simulink model "ctrl_TT_ad_ctrl_cpp_ros_feedback"  (R2022b)
settings: Solver=FixedStepAuto  StartTime=0.0  StopTime=Tf  FixedStep=0.05  RelTol=1e-3
StopFcn:
  | save('testdata')
values from neighbouring files (symbols this model uses):
  adap = 1    [testdata.mat]
  Ba_0 = [0 0 0 0 0 0]    [testdata.mat]
  Bb = 4418825.3321    [testdata.mat]
  Bv_0 = [-5.14444 0 0 0 0 0]    [testdata.mat]
  Bx_0 = [70.34790039 -18.70597267 -370.8000183 0 0 0]    [testdata.mat]
  Cp = [-70.34790039 18.70597267 -370.8000183 -33.25566673 18.72042656 -369.9571533 3.8263092 17.99342728 -368.5174255 40.77630615 14.78142262 -366.2670288 ... (183 elements, 3x61)]    [testdata.mat]    (also in tester.m = [Cpx'; Cpy'; Cpz'])
  Cp_prime = [4.4510680392 0.0017344668 0.1011438 4.44985762706 -0.08575700726 0.1715736104 4.43452754992 -0.37550053768 0.2668049284 4.4276356638 -0.45576590634 0.3213246444 ... (183 elements, 3x61)]    [testdata.mat]
  d = 250    [testdata.mat]
  dA_BP1 = [0.00388591051125 0.00354364911083 0.00553040741788 0.00502167988714 0.0078585088908 0.00748424955325 0.0119232766011 0.0109054787122 0.0168329706434 0.016985509009 0.0156802934897 0.014556760782 ... (616 elements, 616x1)]    [testdata.mat]
  dA_BP2 = [0.00388594063171 0.00354357191533 0.00553040491113 0.00502170939051 0.00785855989083 0.00748435285791 0.0119232653011 0.0109054419481 0.0168329955973 0.0169854794658 0.015680230324 0.0145567225609 ... (616 elements, 616x1)]    [testdata.mat]
  dA_Hull = [0.896301676511 0.898896720864 0.884294141897 0.886832830172 0.870887902011 0.873360353662 0.856223658523 0.858613244346 0.840314828191 0.842595287849 0.823129385532 0.8253007603 ... (2914 elements, 2914x1)]    [testdata.mat]
  dA_PH = [0.00917454029683 0.00917454029683 0.00646521761836 0.00644666811643 0.011728531678 0.0107683420972 0.0165186720105 0.0100399866209 0.0121147162203 0.00917369783051 0.00917369783051 0.00646462373197 ... (550 elements, 550x1)]    [testdata.mat]
  dA_Sail = [0.08073747293 0.0655437895785 0.0678199581962 0.211496702297 0.185444652254 0.10949647106 0.0763960001413 0.0735864235671 0.0440728222699 0.281106392154 0.32735958292 0.104041938486 ... (564 elements, 564x1)]    [testdata.mat]
  dA_SProot = [0.0225345452169 0.0247277274893 0.0225345452169 0.0480467976325 0.0166447079844 0.0410754287554 0.0247277274893 0.0480467976325 0.0468898715351 0.0839833312794 0.0166447079844 0.0255016718 ... (904 elements, 904x1)]    [testdata.mat]
  dA_X1a = [0.0149621011817 0.0166706156701 0.0341149781095 0.0355915100668 0.0512235531199 0.0489176133683 0.0604458424392 0.0503279152264 0.0577124835488 0.0401555322121 0.044833653096 0.0251568218541 ... (200 elements, 200x1)]    [testdata.mat]
  dA_X1b = [0.0149621011817 0.0166706156701 0.0341149781095 0.0355915100668 0.0512235531199 0.0489176133683 0.0604458424392 0.0503279152264 0.0577124835488 0.0401555322121 0.044833653096 0.0251568218541 ... (200 elements, 200x1)]    [testdata.mat]
  dA_X2a = [0.0149620639393 0.0166705502855 0.0341150948266 0.0355913495849 0.051223110376 0.0489180393921 0.0604458270347 0.0503275686692 0.0577128112225 0.0401556683139 0.0448334591683 0.0251566482124 ... (200 elements, 200x1)]    [testdata.mat]
  dA_X2b = [0.0149620639393 0.0166705502855 0.0341150948266 0.0355913495849 0.051223110376 0.0489180393921 0.0604458270347 0.0503275686692 0.0577128112225 0.0401556683139 0.0448334591683 0.0251566482124 ... (200 elements, 200x1)]    [testdata.mat]
  dA_X3a = [0.0149621011817 0.0166706156701 0.0341149781095 0.0355915100668 0.0512235531199 0.0489176133683 0.0604458424392 0.0503279152264 0.0577124835488 0.0401555322121 0.044833653096 0.0251568218541 ... (200 elements, 200x1)]    [testdata.mat]
  dA_X3b = [0.0149621011817 0.0166706156701 0.0341149781095 0.0355915100668 0.0512235531199 0.0489176133683 0.0604458424392 0.0503279152264 0.0577124835488 0.0401555322121 0.044833653096 0.0251568218541 ... (200 elements, 200x1)]    [testdata.mat]
  dA_X4a = [0.0149621011817 0.0166706156701 0.0341149781095 0.0355915100668 0.0512235531199 0.0489176133683 0.0604458424392 0.0503279152264 0.0577124835488 0.0401555322121 0.044833653096 0.0251568218541 ... (200 elements, 200x1)]    [testdata.mat]
  dA_X4b = [0.0149621011817 0.0166706156701 0.0341149781095 0.0355915100668 0.0512235531199 0.0489176133683 0.0604458424392 0.0503279152264 0.0577124835488 0.0401555322121 0.044833653096 0.0251568218541 ... (200 elements, 200x1)]    [testdata.mat]
  Ixx = 52300000    [testdata.mat]
  Ixy = 0    [testdata.mat]
  Ixz = 0    [testdata.mat]
  Iyy = 1375000000    [testdata.mat]
  Iyz = 0    [testdata.mat]
  Izz = 1367000000    [testdata.mat]
  Kp = 0.1    [testdata.mat]
  L1 =     [testdata.mat]
  Mb = 4418825.3321    [testdata.mat]
  n_BP1 = [-0.7747315 -0.03638153 -0.4095958 0 -0.1221389 0 -0.01670914 0 0.005209626 0 0.03404154 0 ... (1848 elements, 616x3)]    [testdata.mat]
  n_BP2 = [-0.774731517 -0.0363815315 -0.409595788 0 -0.122138903 0 -0.0167091396 0 0.00520962616 0 0.0340415388 0 ... (1848 elements, 616x3)]    [testdata.mat]
  n_Hull = [-3.334458e-05 -1.700098e-14 -3.354233e-05 -1.686235e-14 -3.289162e-05 -1.685701e-14 -3.291391e-05 -1.698144e-14 -3.338145e-05 -1.688959e-14 -3.29289e-05 -1.682536e-14 ... (8742 elements, 2914x3)]    [testdata.mat]
  n_PH = [0 0 0.01711651 0.01711627 0.2676807 0.2676804 0.7675173 0.7675174 0.9857236 0 0 0.01711456 ... (1650 elements, 550x3)]    [testdata.mat]
  n_Sail = [-0.05126832 -0.05168081 -0.0485872 -0.03288998 -0.03203588 -0.04435105 -0.04335441 -0.04419429 -0.05169604 0.01094904 0.01649325 -0.03825178 ... (1692 elements, 564x3)]    [testdata.mat]
  n_SProot = [-0.7837688 -0.7969784 -0.7837688 -0.79448 -0.280412 -0.3378876 -0.7969784 -0.79448 -0.7910827 -0.3483897 -0.280412 -0.2790298 ... (2712 elements, 904x3)]    [testdata.mat]
  n_X2a = [-0.283297986 -0.283136904 -0.283195704 -0.28313759 -0.2831586 -0.283137113 -0.28313911 -0.283136606 -0.283121586 -0.283136815 -0.283108413 -0.283138901 ... (600 elements, 200x3)]    [testdata.mat]
  n_X2b = [-0.283297986 -0.283136904 -0.283195704 -0.28313759 -0.2831586 -0.283137113 -0.28313911 -0.283136606 -0.283121586 -0.283136815 -0.283108413 -0.283138901 ... (600 elements, 200x3)]    [testdata.mat]
  n_X3a = [-0.283298 -0.2831369 -0.2831957 -0.2831376 -0.2831586 -0.2831371 -0.2831391 -0.2831366 -0.2831216 -0.2831368 -0.2831084 -0.2831389 ... (600 elements, 200x3)]    [testdata.mat]
  n_X4a = [-0.283298 -0.2831369 -0.2831957 -0.2831376 -0.2831586 -0.2831371 -0.2831391 -0.2831366 -0.2831216 -0.2831368 -0.2831084 -0.2831389 ... (600 elements, 200x3)]    [testdata.mat]
  n_X4b = [-0.283298 -0.2831369 -0.2831957 -0.2831376 -0.2831586 -0.2831371 -0.2831391 -0.2831366 -0.2831216 -0.2831368 -0.2831084 -0.2831389 ... (600 elements, 200x3)]    [testdata.mat]
  nt_BP1 = 616    [testdata.mat]
  nt_BP2 = 616    [testdata.mat]
  nt_Hull = 2914    [testdata.mat]
  nt_PH = 550    [testdata.mat]
  nt_Sail = 564    [testdata.mat]
  nt_SProot = 904    [testdata.mat]
  nt_X1a = 200    [testdata.mat]
  nt_X1b = 200    [testdata.mat]
  nt_X2a = 200    [testdata.mat]
  nt_X2b = 200    [testdata.mat]
  nt_X3a = 200    [testdata.mat]
  nt_X3b = 200    [testdata.mat]
  nt_X4a = 200    [testdata.mat]
  nt_X4b = 200    [testdata.mat]
  Seastate = 0    [testdata.mat]
  Tf = 500    [testdata.mat]    (also in tester.m)
  Ts = 0.05    [testdata.mat]
  vt1_BP1 = [-11.0524049722 -10.9924120522 -10.9924120522 -10.8819663922 -10.8819663922 -10.7297166322 -10.7297166322 -10.5070632922 -10.5070632922 -10.1807245522 -10.1807245522 -9.8815181122 ... (1848 elements, 616x3)]    [testdata.mat]
  vt1_BP2 = [-11.0524048318 -10.9924111396 -10.9924111396 -10.8819658306 -10.8819658306 -10.7297157898 -10.7297157898 -10.5070637134 -10.5070637134 -10.1807238502 -10.1807238502 -9.8815188844 ... (1848 elements, 616x3)]    [testdata.mat]
  vt1_Hull = [3.5122487678 3.7304022878 5.2621803278 5.4863499878 6.9866994878 7.2167238278 8.6832650078 8.9189474678 10.3493567078 10.5904445678 11.9823842078 12.2286247478 ... (8742 elements, 2914x3)]    [testdata.mat]
  vt1_PH = [37.3342788278 37.3342788278 37.4268866678 37.4268866678 37.5892452278 37.5892452278 37.7549453078 37.7549453078 37.8074619278 37.3342788278 37.3342788278 37.4268866678 ... (1650 elements, 550x3)]    [testdata.mat]
  vt1_Sail = [-12.4909433722 -12.1578443722 -12.0399645322 -11.2138368922 -10.6240515922 -11.5111900522 -11.9364967522 -11.6561249722 -12.4909433722 -7.5732648922 -6.8453119522 -11.1890071522 ... (1692 elements, 564x3)]    [testdata.mat]
  vt1_SProot = [29.2099766678 29.1371231078 29.0494854278 29.2099766678 29.2862630078 29.4526510478 29.0494854278 29.1261368078 29.3369263478 29.5706712878 29.0494854278 29.3857364078 ... (2712 elements, 904x3)]    [testdata.mat]
  vt1_X1a = [29.3961751478 29.4776282078 29.4776282078 29.7060309278 29.7060309278 30.0693861278 30.0693861278 30.5458756478 30.5458756478 31.0830460478 31.0830460478 31.6023926678 ... (600 elements, 200x3)]    [testdata.mat]
  vt1_X1b = [29.6638337078 29.6638337078 29.9620713878 29.9620713878 30.3181187678 30.3181187678 30.7116389078 30.7116389078 31.1104380878 31.1104380878 31.4810519678 31.4810519678 ... (600 elements, 200x3)]    [testdata.mat]
  vt1_X2a = [29.3961767624 29.4776272952 29.4776272952 29.7060326828 29.7060326828 30.0693842324 30.0693842324 30.5458736822 30.5458736822 31.083047171 31.083047171 31.6023916148 ... (600 elements, 200x3)]    [testdata.mat]
  vt1_X2b = [29.6638345502 29.6638345502 29.9620708964 29.9620708964 30.3181168022 30.3181168022 30.7116409436 30.7116409436 31.1104372454 31.1104372454 31.4810526698 31.4810526698 ... (600 elements, 200x3)]    [testdata.mat]
  vt1_X3a = [29.3961751478 29.4776282078 29.4776282078 29.7060309278 29.7060309278 30.0693861278 30.0693861278 30.5458756478 30.5458756478 31.0830460478 31.0830460478 31.6023926678 ... (600 elements, 200x3)]    [testdata.mat]
  vt1_X3b = [29.6638337078 29.6638337078 29.9620713878 29.9620713878 30.3181187678 30.3181187678 30.7116389078 30.7116389078 31.1104380878 31.1104380878 31.4810519678 31.4810519678 ... (600 elements, 200x3)]    [testdata.mat]
  vt1_X4a = [29.6638337078 29.6638337078 29.9620713878 29.9620713878 30.3181187678 30.3181187678 30.7116389078 30.7116389078 31.1104380878 31.1104380878 31.4810519678 31.4810519678 ... (600 elements, 200x3)]    [testdata.mat]
  vt1_X4b = [29.3961751478 29.4776282078 29.4776282078 29.7060309278 29.7060309278 30.0693861278 30.0693861278 30.5458756478 30.5458756478 31.0830460478 31.0830460478 31.6023926678 ... (600 elements, 200x3)]    [testdata.mat]
  vt2_BP1 = [-10.9924120522 -10.9494777322 -10.8819663922 -10.8505308322 -10.7297166322 -10.7112259522 -10.5070632922 -10.4997203722 -10.1807245522 -10.1757543922 -9.8815181122 -9.8813004922 ... (1848 elements, 616x3)]    [testdata.mat]
  vt2_BP2 = [-11.0294626294 -11.0294626294 -10.9494786448 -10.9494786448 -10.8505316746 -10.8505316746 -10.7112256012 -10.7112256012 -10.499720302 -10.499720302 -10.1757550942 -10.1757550942 ... (1848 elements, 616x3)]    [testdata.mat]
  vt2_Hull = [1.9517168078 1.9517168078 3.7304022878 3.7304022878 5.4863499878 5.4863499878 7.2167238278 7.2167238278 8.9189474678 8.9189474678 10.5904445678 10.5904445678 ... (8742 elements, 2914x3)]    [testdata.mat]
  vt2_PH = [37.2028433678 37.2028433678 37.3342788278 37.4268866678 37.4268866678 37.5892452278 37.5892452278 37.7549453078 37.7549453078 37.2028433678 37.2028433678 37.3342788278 ... (1650 elements, 550x3)]    [testdata.mat]
  vt2_Sail = [-12.0399645322 -12.0399645322 -11.9364967522 -10.7084881522 -10.7084881522 -12.0399645322 -12.0399645322 -11.9364967522 -12.3734566522 -7.7110323922 -7.7110323922 -11.6561249722 ... (1692 elements, 564x3)]    [testdata.mat]
  vt2_SProot = [29.0494854278 29.0494854278 29.2099766678 29.1261368078 29.0494854278 29.1371231078 29.1371231078 29.2099766678 29.1261368078 29.2099766678 29.2862630078 29.2862630078 ... (2712 elements, 904x3)]    [testdata.mat]
  vt2_X1a = [29.4776282078 29.9620713878 29.7060309278 30.3181187678 30.0693861278 30.7116389078 30.5458756478 31.1104380878 31.0830460478 31.4810519678 31.6023926678 31.7970362078 ... (600 elements, 200x3)]    [testdata.mat]
  vt2_X1b = [29.4776282078 29.9620713878 29.7060309278 30.3181187678 30.0693861278 30.7116389078 30.5458756478 31.1104380878 31.0830460478 31.4810519678 31.6023926678 31.7970362078 ... (600 elements, 200x3)]    [testdata.mat]
  vt2_X2a = [29.6638345502 29.6638345502 29.9620708964 29.9620708964 30.3181168022 30.3181168022 30.7116409436 30.7116409436 31.1104372454 31.1104372454 31.4810526698 31.4810526698 ... (600 elements, 200x3)]    [testdata.mat]
  vt2_X2b = [29.3961767624 29.4776272952 29.4776272952 29.7060326828 29.7060326828 30.0693842324 30.0693842324 30.5458736822 30.5458736822 31.083047171 31.083047171 31.6023916148 ... (600 elements, 200x3)]    [testdata.mat]
  vt2_X3a = [29.4776282078 29.9620713878 29.7060309278 30.3181187678 30.0693861278 30.7116389078 30.5458756478 31.1104380878 31.0830460478 31.4810519678 31.6023926678 31.7970362078 ... (600 elements, 200x3)]    [testdata.mat]
  vt2_X3b = [29.4776282078 29.9620713878 29.7060309278 30.3181187678 30.0693861278 30.7116389078 30.5458756478 31.1104380878 31.0830460478 31.4810519678 31.6023926678 31.7970362078 ... (600 elements, 200x3)]    [testdata.mat]
  vt2_X4a = [29.4776282078 29.9620713878 29.7060309278 30.3181187678 30.0693861278 30.7116389078 30.5458756478 31.1104380878 31.0830460478 31.4810519678 31.6023926678 31.7970362078 ... (600 elements, 200x3)]    [testdata.mat]
  vt2_X4b = [29.4776282078 29.9620713878 29.7060309278 30.3181187678 30.0693861278 30.7116389078 30.5458756478 31.1104380878 31.0830460478 31.4810519678 31.6023926678 31.7970362078 ... (600 elements, 200x3)]    [testdata.mat]
  vt3_BP1 = [-11.0294636122 -11.0294636122 -10.9494777322 -10.9494777322 -10.8505308322 -10.8505308322 -10.7112259522 -10.7112259522 -10.4997203722 -10.4997203722 -10.1757543922 -10.1757543922 ... (1848 elements, 616x3)]    [testdata.mat]
  vt3_BP2 = [-10.9924111396 -10.9494786448 -10.8819658306 -10.8505316746 -10.7297157898 -10.7112256012 -10.5070637134 -10.499720302 -10.1807238502 -10.1757550942 -9.8815188844 -9.8813013346 ... (1848 elements, 616x3)]    [testdata.mat]
  vt3_Hull = [1.7397198278 3.5122487678 3.5122487678 5.2621803278 5.2621803278 6.9866994878 6.9866994878 8.6832650078 8.6832650078 10.3493567078 10.3493567078 11.9823842078 ... (8742 elements, 2914x3)]    [testdata.mat]
  vt3_PH = [37.2028433678 37.3342788278 37.3342788278 37.3342788278 37.4268866678 37.4268866678 37.5892452278 37.5892452278 37.7549453078 37.2028433678 37.3342788278 37.3342788278 ... (1650 elements, 550x3)]    [testdata.mat]
  vt3_Sail = [-12.3734566522 -12.4909433722 -12.3734566522 -11.5111900522 -11.2138368922 -11.7698559922 -11.5111900522 -11.5111900522 -12.1578443722 -8.3109054322 -7.5732648922 -11.5111900522 ... (1692 elements, 564x3)]    [testdata.mat]
  vt3_SProot = [29.1261368078 29.2099766678 29.1261368078 29.3369263478 29.1371231078 29.2099766678 29.2099766678 29.3369263478 29.2548344678 29.3369263478 29.1371231078 29.1371231078 ... (2712 elements, 904x3)]    [testdata.mat]
  vt3_X1a = [29.6638337078 29.6638337078 29.9620713878 29.9620713878 30.3181187678 30.3181187678 30.7116389078 30.7116389078 31.1104380878 31.1104380878 31.4810519678 31.4810519678 ... (600 elements, 200x3)]    [testdata.mat]
  vt3_X1b = [29.3961751478 29.4776282078 29.4776282078 29.7060309278 29.7060309278 30.0693861278 30.0693861278 30.5458756478 30.5458756478 31.0830460478 31.0830460478 31.6023926678 ... (600 elements, 200x3)]    [testdata.mat]
  vt3_X2a = [29.4776272952 29.9620708964 29.7060326828 30.3181168022 30.0693842324 30.7116409436 30.5458736822 31.1104372454 31.083047171 31.4810526698 31.6023916148 31.7970343826 ... (600 elements, 200x3)]    [testdata.mat]
  vt3_X2b = [29.4776272952 29.9620708964 29.7060326828 30.3181168022 30.0693842324 30.7116409436 30.5458736822 31.1104372454 31.083047171 31.4810526698 31.6023916148 31.7970343826 ... (600 elements, 200x3)]    [testdata.mat]
  vt3_X3a = [29.6638337078 29.6638337078 29.9620713878 29.9620713878 30.3181187678 30.3181187678 30.7116389078 30.7116389078 31.1104380878 31.1104380878 31.4810519678 31.4810519678 ... (600 elements, 200x3)]    [testdata.mat]
  vt3_X3b = [29.3961751478 29.4776282078 29.4776282078 29.7060309278 29.7060309278 30.0693861278 30.0693861278 30.5458756478 30.5458756478 31.0830460478 31.0830460478 31.6023926678 ... (600 elements, 200x3)]    [testdata.mat]
  vt3_X4a = [29.3961751478 29.4776282078 29.4776282078 29.7060309278 29.7060309278 30.0693861278 30.0693861278 30.5458756478 30.5458756478 31.0830460478 31.0830460478 31.6023926678 ... (600 elements, 200x3)]    [testdata.mat]
  vt3_X4b = [29.6638337078 29.6638337078 29.9620713878 29.9620713878 30.3181187678 30.3181187678 30.7116389078 30.7116389078 31.1104380878 31.1104380878 31.4810519678 31.4810519678 ... (600 elements, 200x3)]    [testdata.mat]
  Xb = 0    [testdata.mat]
  Xcg = [32.3287332922 0 0]    [testdata.mat]
  Xg = 0    [testdata.mat]
  Yb = 0    [testdata.mat]
  Yg = 0    [testdata.mat]
  Zb = 0.4406    [testdata.mat]
  Zg = 0    [testdata.mat]
libraries: robotlib x54, simulink x8, sharedtransform x2, dspmathops x2
(part 3 of 9)

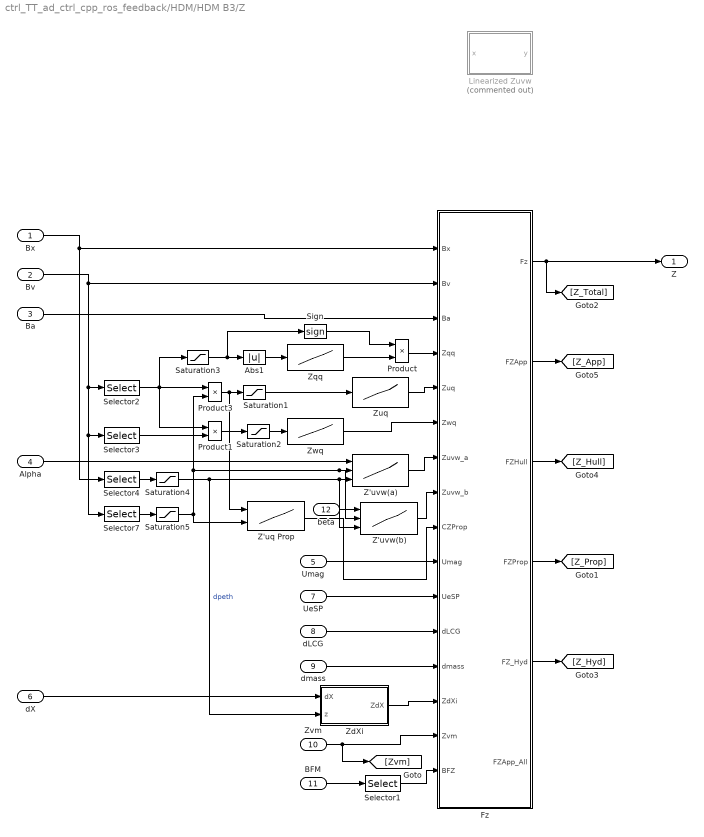
== system ctrl_TT_ad_ctrl_cpp_ros_feedback/HDM/HDM B3/Z ==
  Bx : Inport
  Bv : Inport  Port=2
  Ba : Inport  Port=3
  Alpha : Inport  Port=4
  Umag : Inport  Port=5
  dX : Inport  Port=6
  UeSP : Inport  Port=7
  dLCG : Inport  Port=8
  dmass : Inport  Port=9
  Zvm : Inport  Port=10
  BFM : Inport  Port=11
  beta : Inport  Port=12
  Abs1 : Abs  SaturateOnIntegerOverflow=off
  Fz : MATLAB Function  TreatAsAtomicUnit=on
  Linearized Zuvw : MATLAB Function  Commented=on  TreatAsAtomicUnit=on
  Product : Product
  Product1 : Product
  Product3 : Product
  Saturation1 : Saturate  UpperLimit=0.04  LowerLimit=-0.04
  Saturation2 : Saturate  UpperLimit=0.0015  LowerLimit=-0.0015
  Saturation3 : Saturate  UpperLimit=0.02  LowerLimit=-0.02
  Saturation4 : Saturate  UpperLimit=-13.8724  LowerLimit=-35.0624
  Saturation5 : Saturate  UpperLimit=-1.5433E+00  LowerLimit=-5.14444
  Selector1 : Selector  InputPortWidth=6  IndexOptions=Index vector (dialog)  Indices=3  OutputSizes=1
  Selector2 : Selector  InputPortWidth=6  IndexOptions=Index vector (dialog)  Indices=5  OutputSizes=1
  Selector3 : Selector  InputPortWidth=6  IndexOptions=Index vector (dialog)  Indices=3  OutputSizes=1
  Selector4 : Selector  InputPortWidth=6  IndexOptions=Index vector (dialog)  Indices=3  OutputSizes=1
  Selector7 : Selector  InputPortWidth=6  IndexOptions=Index vector (dialog)  Indices=1  OutputSizes=1
  Sign : Signum
  Z'uq Prop : Lookup_n-D  BreakpointsForDimension1=|  BreakpointsForDimension2=[-7.71666 -5.14444 -3.086664 -1.543332]  Table=|  InternalRulePriority=Speed  RndMeth=Simplest
      BreakpointsForDimension1=|
      | [-2.0E-01
      | -1.5E-01
      | -1.0E-01
      | -5.0E-02
      | 0.0E+00
      | 5.0E-02
      | 1.0E-01
      | 1.5E-01
      | 2.0E-01
      | ]
      Table=|
      | reshape([1.3913E-04
      | 1.0452E-04
      | 6.9900E-05
      | 3.5283E-05
      | 6.6700E-07
      | -3.3949E-05
      | -6.8566E-05
      | -1.0318E-04
      | -1.3780E-04
      | 2.8914E-04
      | 2.1702E-04
      | 1.4490E-04
      | 7.2785E-05
      | 6.6700E-07
      | -7.1451E-05
      | -1.4357E-04
      | -2.1569E-04
      | -2.8780E-04
      | 1.1606E-04
      | 8.7208E-05
      | 5.8361E-05
      | 2.9514E-05
      | 6.6700E-07
      | -2.8180E-05
      | -5.7027E-05
      | -8.5874E-05
      | -1.1472E-04
      | 1.1606E-04
      | 8.7208E-05
      | 5.8361E-05
      | 2.9514E-05
      | 6.6700E-07
      | -2.8180E-05
      | -5.7027E-05
      | -8.5874E-05
      | -1.1472E-04],[9,4])
      settings: InputPortMap=u0,u1
  Z'uvw(a) : Lookup_n-D  NumberOfTableDimensions=3  BreakpointsForDimension1=|  BreakpointsForDimension2=|  BreakpointsForDimension3=|  Table=|  InternalRulePriority=Speed  RndMeth=Simplest
      BreakpointsForDimension1=|
      | [-12
      | -8
      | -4
      | 0
      | 4
      | 8
      | 12]
      BreakpointsForDimension2=|
      | [-5.1444E+00
      | -3.0866E+00
      | -1.5433E+00
      | ]
      Table=|
      | reshape([-3.82587E-03
      | -2.42543E-03
      | -1.05453E-03
      | 1.94202E-04
      | 1.48991E-03
      | 3.04047E-03
      | 4.14104E-03
      | -3.76348E-03
      | -2.38508E-03
      | -9.82619E-04
      | 1.94202E-04
      | 1.47560E-03
      | 3.02863E-03
      | 4.06663E-03
      | -3.75964E-03
      | -2.29001E-03
      | -8.34074E-04
      | 1.94202E-04
      | 1.38956E-03
      | 2.91153E-03
      | 4.15251E-03
      | -3.11218E-03
      | -1.80502E-03
      | -4.97855E-04
      | 8.09305E-04
      | 2.11647E-03
      | 3.42363E-03
      | 4.73079E-03
      | -2.62573E-03
      | -1.48072E-03
      | -3.35708E-04
      | 8.09305E-04
      | 1.95432E-03
      | 3.09933E-03
      | 4.24434E-03
      | -2.06413E-03
      | -1.10632E-03
      | -1.48507E-04
      | 8.09305E-04
      | 1.76712E-03
      | 2.72493E-03
      | 3.68274E-03
      | -3.09997E-03
      | -1.76300E-03
      | -4.26025E-04
      | 9.10947E-04
      | 2.24792E-03
      | 3.58489E-03
      | 4.92186E-03
      | -2.49055E-03
      | -1.35672E-03
      | -2.22886E-04
      | 9.10947E-04
      | 2.04478E-03
      | 3.17861E-03
      | 4.31245E-03
      | -2.64104E-03
      | -1.45704E-03
      | -2.73048E-04
      | 9.10947E-04
      | 2.09494E-03
      | 3.27894E-03
      | 4.46293E-03
      | -0.003059752
      | -0.001711935
      | -0.000364117
      | 0.0009837
      | 0.002331518
      | 0.003679335
      | 0.005027153
      | -0.002351082
      | -0.0012256
      | -0.000100118
      | 0.0009837
      | 0.002109182
      | 0.003234664
      | 0.004360146
      | -0.001725739
      | -0.000822593
      | 8.05539E-05
      | 0.0009837
      | 0.001886847
      | 0.002789993
      | 0.00369314],[7,3,4])
      BreakpointsForDimension3=|
      | [-35.0624 -18.3724 -15.3724 -13.8724
      | ]
      settings: InputPortMap=u0,u1,u2
  Z'uvw(b) : Lookup_n-D  NumberOfTableDimensions=3  BreakpointsForDimension1=|  BreakpointsForDimension2=|  BreakpointsForDimension3=|  Table=|  InternalRulePriority=Speed  RndMeth=Simplest
      BreakpointsForDimension1=|
      | [0
      | 4
      | 8
      | 12]
      BreakpointsForDimension2=|
      | [-5.1444E+00
      | -3.0866E+00
      | -1.5433E+00
      | ]
      Table=|
      | reshape([0.0000000E+00
      | -5.9986916E-04
      | -2.7503348E-03
      | -5.0777589E-03
      | 0.0000000E+00
      | -6.0654884E-04
      | -2.4512564E-03
      | -5.2464901E-03
      | 0.0000000E+00
      | -7.6137528E-04
      | -2.4084463E-03
      | -5.2118678E-03
      | 0.0000000E+00
      | -8.2427914E-04
      | -2.5250249E-03
      | -5.3103563E-03
      | 0.0000000E+00
      | -8.1036019E-04
      | -2.5315266E-03
      | -5.5141459E-03
      | 0.0000000E+00
      | -7.9799041E-04
      | -2.5595242E-03
      | -5.2319004E-03
      | 0.0000000E+00
      | -8.6989011E-04
      | -2.5865820E-03
      | -5.6151595E-03
      | 0.0000000E+00
      | -8.4361582E-04
      | -2.6124115E-03
      | -5.7143353E-03
      | 0.0000000E+00
      | -8.2567611E-04
      | -2.6088331E-03
      | -5.6150660E-03
      | 0.0000000E+00
      | -9.1003224E-04
      | -2.7683191E-03
      | -6.0189061E-03
      | 0.0000000E+00
      | -8.4211433E-04
      | -2.5899187E-03
      | -5.7497784E-03
      | 0.0000000E+00
      | -8.2014014E-04
      | -2.4092466E-03
      | -5.6643347E-03],[4,3,4])
      BreakpointsForDimension3=|
      | [-35.0624 -18.3724 -15.3724 -13.8724
      | ]
      settings: InputPortMap=u0,u1,u2
  ZdXi : Subsystem
  Zqq : Lookup_n-D  NumberOfTableDimensions=1  BreakpointsForDimension1=|  Table=|  InternalRulePriority=Speed  RndMeth=Simplest
      BreakpointsForDimension1=|
      | [0.000127901
      | 0.000383704
      | 0.000639507
      | 0.001279013
      | 0.002558026
      | ]
      Table=|
      | [-1.5611E-03
      | -1.0379E-04
      | 3.9238E-05
      | 1.1475E-04
      | 1.3579E-04
      | ]
  Zuq : Lookup_n-D  NumberOfTableDimensions=1  BreakpointsForDimension1=|  Table=|  InternalRulePriority=Speed  RndMeth=Simplest
      BreakpointsForDimension1=|
      | [-0.04
      | -0.03
      | -0.02
      | -0.01
      | -0.005
      | -0.002
      | 0.002
      | 0.005
      | 0.01
      | 0.02
      | 0.03
      | 0.04
      | ]
      Table=|
      | [-9.8908E-03
      | -9.0784E-03
      | -8.9566E-03
      | -1.0733E-02
      | -1.4141E-02
      | -2.4189E-02
      | -6.5605E-03
      | -7.1594E-03
      | -7.6366E-03
      | -7.9008E-03
      | -6.1794E-03
      | -6.1029E-03
      | ]
  Zwq : Lookup_n-D  NumberOfTableDimensions=1  BreakpointsForDimension1=|  Table=|  InternalRulePriority=Speed  RndMeth=Simplest
      BreakpointsForDimension1=|
      | [-0.0015
      | -0.0012
      | -0.0009
      | -0.0006
      | -0.0003
      | -0.0001
      | 0.0001
      | 0.0003
      | 0.0006
      | 0.0009
      | 0.0012
      | 0.0015]
      Table=|
      | [-2.9784E-01
      | -2.6725E-01
      | -2.3292E-01
      | -2.0077E-01
      | -1.1489E-01
      | -7.6673E-03
      | -7.5516E-03
      | -1.1617E-01
      | -2.0077E-01
      | -2.9128E-01
      | -3.5974E-01
      | -4.7839E-01]
  Z : Outport
  wires:
  beta/1 -> Z'uvw(b)/1
  Z'uvw(b)/1 -> Fz/8(Zuvw_b)
  Product/1 -> Fz/4(Zqq)
  Sign/1 -> Product/1
  Abs1/1 -> Zqq/1
  Selector7/1 -> Saturation5/1
  Saturation5/1 -> Z'uq Prop/2, Z'uvw(b)/2, Z'uvw(a)/2, Product3/2
  Saturation4/1 -> ZdXi/2(z), Z'uvw(a)/3, Z'uvw(b)/3  "dpeth"
  Fz/5(FZ_Hyd) -> [Z_Hyd]
  Fz/4(FZProp) -> [Z_Prop]
  Fz/3(FZHull) -> [Z_Hull]
  Fz/2(FZApp) -> [Z_App]
  ZdXi/1(ZdX) -> Fz/14(ZdXi)
  Selector1/1 -> Fz/16(BFZ)
  BFM/1 -> Selector1/1
  Z'uvw(a)/1 -> Fz/7(Zuvw_a)
  Zqq/1 -> Product/2
  Z'uq Prop/1 -> Fz/9(CZProp)
  Zwq/1 -> Fz/6(Zwq)
  Selector2/1 -> Saturation3/1, Product1/1, Product3/1
  Alpha/1 -> Z'uvw(a)/1
  Bv/1 -> Selector7/1, Selector3/1, Selector2/1, Fz/2(Bv)
  Umag/1 -> Fz/10(Umag)
  Bx/1 -> Selector4/1, Fz/1(Bx)
  Product3/1 -> Z'uq Prop/1, Saturation1/1
  UeSP/1 -> Fz/11(UeSP)
  Selector3/1 -> Product1/2
  Product1/1 -> Saturation2/1
  dLCG/1 -> Fz/12(dLCG)
  dmass/1 -> Fz/13(dmass)
  dX/1 -> ZdXi/1(dX)
  Saturation1/1 -> Zuq/1
  Saturation2/1 -> Zwq/1
  Saturation3/1 -> Sign/1, Abs1/1
  Fz/1(Fz) -> [Z_Total], Z/1
  Zuq/1 -> Fz/5(Zuq)
  Ba/1 -> Fz/3(Ba)
  Zvm/1 -> [Zvm], Fz/15(Zvm)
  Selector4/1 -> Saturation4/1

== system ctrl_TT_ad_ctrl_cpp_ros_feedback/HDM/Integration and Coord. Transfrom/Coordinate Transform ==
  Bv : Inport
  Integrator : Integrator  InitialCondition=Bx_0
  MATLAB Function2 : MATLAB Function  TreatAsAtomicUnit=on
  X_earth : Outport  VectorParamsAs1DForOutWhenUnconnected=off
  wires:
  MATLAB Function2/1(out) -> Integrator/1
  Bv/1 -> MATLAB Function2/2(Bv)
  Integrator/1 -> X_earth/1, MATLAB Function2/1(Bx)

== system ctrl_TT_ad_ctrl_cpp_ros_feedback/HDM/Integration and Coord. Transfrom/Rigid Body Motion ==
  F_hyd : Inport
  Bx : Inport  Port=2
  Demux : Demux  Outputs=6
  Demux1 : Demux  Outputs=6
  Demux2 : Demux  Outputs=5
  Gain2 : Gain
  Integrator : Integrator  InitialCondition=Bv_0
  MATLAB Function2 : MATLAB Function  TreatAsAtomicUnit=on
  Memory1 : Memory  InitialCondition=Ba_0
  Mux1 : Mux  Inputs=6
  Mux2 : Mux  Inputs=5
  Bv : Outport  VectorParamsAs1DForOutWhenUnconnected=off
  Ba : Outport  Port=2  VectorParamsAs1DForOutWhenUnconnected=off
  wires:
  Mux1/1 -> Bv/1
  Gain2/1 -> Demux2/1
  Demux1/2 -> Mux2/1
  Demux1/4 -> Mux2/3
  Demux1/6 -> Mux2/5
  Demux1/5 -> Mux2/4
  Demux2/1 -> Mux1/2
  Demux1/1 -> Mux1/1
  Demux2/4 -> Mux1/5
  Demux2/2 -> Mux1/3
  Demux2/5 -> Mux1/6
  Mux2/1 -> Gain2/1
  Demux1/3 -> Mux2/2
  Demux2/3 -> Mux1/4
  F_hyd/1 -> Demux/1
  Demux/6 -> MATLAB Function2/6(N)
  Demux/5 -> MATLAB Function2/5(M)
  Demux/4 -> MATLAB Function2/4(K)
  Demux/3 -> MATLAB Function2/3(Z)
  Demux/2 -> MATLAB Function2/2(Y)
  Demux/1 -> MATLAB Function2/1(X)
  Memory1/1 -> Ba/1
  Integrator/1 -> Demux1/1, MATLAB Function2/8(bv)
  MATLAB Function2/1(out) -> Memory1/1, Integrator/1
  Bx/1 -> MATLAB Function2/7(bx)

== system ctrl_TT_ad_ctrl_cpp_ros_feedback/HDM/actuator saturation/  ==
  "dX " : Inport
  Constant{,3,5,7,9} (5 alike) : Constant  Value=7.11
  Constant{2,4,6,8,10} (5 alike) : Constant  Value=-7.11
  Demux3 : Demux  Outputs=5
  I-Pitch{1..5} (5 alike) : Gain
  Max Deflection{,1..4} (5 alike) : Saturate  UpperLimit=30  LowerLimit=-30
  Mux : Mux  Inputs=5
  Rate Limiter Dynamic{,1..4} (5 alike) : simulink/Discontinuities/Rate Limiter Dynamic
  Scope : Scope  NumInputPorts=5
  dX : Outport
  wires:
  Rate Limiter Dynamic3/1 -> Max Deflection3/1
  Mux/1 -> dX/1
  Constant7/1 -> Rate Limiter Dynamic3/1
  Max Deflection4/1 -> I-Pitch5/1  "dV"
  Constant8/1 -> Rate Limiter Dynamic3/3
  "dX "/1 -> Demux3/1
  Max Deflection3/1 -> I-Pitch4/1  "dV"
  Constant5/1 -> Rate Limiter Dynamic2/1
  Max Deflection1/1 -> I-Pitch1/1  "dV"
  Rate Limiter Dynamic2/1 -> Max Deflection2/1
  Constant/1 -> Rate Limiter Dynamic/1
  Rate Limiter Dynamic1/1 -> Max Deflection1/1
  Constant6/1 -> Rate Limiter Dynamic2/3
  I-Pitch4/1 -> Mux/4, Scope/4
  I-Pitch3/1 -> Mux/1, Scope/1
  Constant4/1 -> Rate Limiter Dynamic1/3
  I-Pitch1/1 -> Mux/2, Scope/2
  Max Deflection2/1 -> I-Pitch2/1  "dV"
  Rate Limiter Dynamic4/1 -> Max Deflection4/1
  I-Pitch5/1 -> Mux/5, Scope/5
  Rate Limiter Dynamic/1 -> Max Deflection/1
  Constant10/1 -> Rate Limiter Dynamic4/3
  Demux3/2 -> Rate Limiter Dynamic1/2
  Demux3/4 -> Rate Limiter Dynamic3/2
  Constant3/1 -> Rate Limiter Dynamic1/1
  Demux3/5 -> Rate Limiter Dynamic4/2
  Demux3/3 -> Rate Limiter Dynamic2/2
  Max Deflection/1 -> I-Pitch3/1  "dV"
  Demux3/1 -> Rate Limiter Dynamic/2
  Constant9/1 -> Rate Limiter Dynamic4/1
  Constant2/1 -> Rate Limiter Dynamic/3
  I-Pitch2/1 -> Mux/3, Scope/3

== system ctrl_TT_ad_ctrl_cpp_ros_feedback/HDM/actuator saturation/    ==
  "n " : Inport
  Rate Limiter Dynamic : simulink/Discontinuities/Rate Limiter Dynamic
  Rate Max : Constant  Value=14.65
  Rate Min : Constant  Value=-14.65
  Saturation6 : Saturate  UpperLimit=10  LowerLimit=0.01
  n : Outport
  wires:
  Saturation6/1 -> n/1
  Rate Max/1 -> Rate Limiter Dynamic/1
  Rate Limiter Dynamic/1 -> Saturation6/1
  Rate Min/1 -> Rate Limiter Dynamic/3
  "n "/1 -> Rate Limiter Dynamic/2

== system ctrl_TT_ad_ctrl_cpp_ros_feedback/HDM/actuator saturation/Subsystem1 ==
  dLCG : Inport
  " LCG Change Saturation" : Saturate
  Lower Rate limit : Constant  Value=-5.83e-4
  Rate Limiter Dynamic : simulink/Discontinuities/Rate Limiter Dynamic
  Upper Rate limit : Constant  Value=5.83e-4
  dLCG (m) : Outport
  wires:
  dLCG/1 -> Rate Limiter Dynamic/2
  Upper Rate limit/1 -> Rate Limiter Dynamic/1
  Lower Rate limit/1 -> Rate Limiter Dynamic/3
  Rate Limiter Dynamic/1 -> " LCG Change Saturation"/1  "dLCG (m)"
  " LCG Change Saturation"/1 -> dLCG (m)/1  "dLCG (m)"

== system ctrl_TT_ad_ctrl_cpp_ros_feedback/HDM/actuator saturation/Subsystem2 ==
  dmass : Inport
  Constant2 : Constant  Value=100
  Constant3 : Constant  Value=-100
  Max Mass Change : Saturate  UpperLimit=20000  LowerLimit=-20000
  Rate Limiter Dynamic1 : simulink/Discontinuities/Rate Limiter Dynamic
  dmass (kg) : Outport
  wires:
  Max Mass Change/1 -> dmass (kg)/1  "dmass (kg)"
  dmass/1 -> Rate Limiter Dynamic1/2
  Constant2/1 -> Rate Limiter Dynamic1/1
  Rate Limiter Dynamic1/1 -> Max Mass Change/1  "dmass (kg)"
  Constant3/1 -> Rate Limiter Dynamic1/3

== system ctrl_TT_ad_ctrl_cpp_ros_feedback/HDM/HDM B3/K/KdXi ==
  dX : Inport
  UeX : Inport  Port=2
  z : Inport  Port=3
  KdX1 : Lookup_n-D  NumberOfTableDimensions=3  BreakpointsForDimension1=[-10 0 10]  BreakpointsForDimension2=|  BreakpointsForDimension3=[-5.14444 -3.08666664 -1.54332]  Table=|  InternalRulePriority=Speed  RndMeth=Simplest
      BreakpointsForDimension2=|
      | [-36.4062987
      | -18.4062987
      | -15.4062987
      | -13.9062987]
      Table=|
      | reshape([-3.9047E-05
      | 4.5684E-07
      | 3.9769E-05
      | -3.8309E-05
      | 1.2643E-06
      | 4.0809E-05
      | -3.0256E-05
      | 1.2643E-06
      | 4.8387E-05
      | -3.7558E-05
      | 2.1545E-06
      | 4.2083E-05
      | -3.9057E-05
      | 3.6064E-07
      | 3.9562E-05
      | -3.8473E-05
      | 1.0476E-06
      | 4.0437E-05
      | -3.0256E-05
      | 1.4418E-06
      | 4.8387E-05
      | -3.7906E-05
      | 1.7415E-06
      | 4.1434E-05
      | -3.8945E-05
      | 2.8249E-07
      | 3.9429E-05
      | -3.8396E-05
      | 9.1134E-07
      | 4.0237E-05
      | -3.8190E-05
      | 9.1134E-07
      | 4.0733E-05
      | -3.7932E-05
      | 1.5343E-06
      | 4.1020E-05
      | ],[3,4,3])
      settings: InputPortMap=u0,u1,u2
  KdX2 : Lookup_n-D  NumberOfTableDimensions=3  BreakpointsForDimension1=[-10 0 10]  BreakpointsForDimension2=|  BreakpointsForDimension3=[-5.14444 -3.08666664 -1.54332]  Table=|  InternalRulePriority=Speed  RndMeth=Simplest
      BreakpointsForDimension2=|
      | [-36.4062987
      | -18.4062987
      | -15.4062987
      | -13.9062987]
      Table=|
      | reshape([-3.5775E-05
      | -2.4080E-07
      | 3.3150E-05
      | -3.4263E-05
      | 1.2268E-06
      | 3.5342E-05
      | -2.3577E-05
      | 1.2268E-06
      | 4.6338E-05
      | -3.2368E-05
      | 3.5682E-06
      | 3.9469E-05
      | -3.5785E-05
      | -3.3131E-07
      | 3.3067E-05
      | -3.4544E-05
      | 8.9010E-07
      | 3.4889E-05
      | -2.3577E-05
      | 1.7076E-06
      | 4.6338E-05
      | -3.3141E-05
      | 2.4187E-06
      | 3.7389E-05
      | -3.5809E-05
      | -5.7189E-07
      | 3.3046E-05
      | -3.4706E-05
      | 4.2723E-07
      | 3.4588E-05
      | -3.4017E-05
      | 4.2723E-07
      | 3.5657E-05
      | -3.3562E-05
      | 1.6134E-06
      | 3.6605E-05
      | ],[3,4,3])
      settings: InputPortMap=u0,u1,u2
  KdX3 : Lookup_n-D  NumberOfTableDimensions=3  BreakpointsForDimension1=[-10 0 10]  BreakpointsForDimension2=|  BreakpointsForDimension3=[-5.14444 -3.08666664 -1.54332]  Table=|  InternalRulePriority=Speed  RndMeth=Simplest
      BreakpointsForDimension2=|
      | [-36.4062987
      | -18.4062987
      | -15.4062987
      | -13.9062987]
      Table=|
      | reshape([-4.3139E-05
      | 1.7292E-07
      | 4.5001E-05
      | -4.4081E-05
      | -1.2796E-06
      | 4.2448E-05
      | -4.9749E-05
      | -1.2796E-06
      | 2.6691E-05
      | -4.5613E-05
      | -3.5861E-06
      | 3.8362E-05
      | -4.2707E-05
      | 2.7384E-07
      | 4.4575E-05
      | -4.3360E-05
      | -9.3523E-07
      | 4.2465E-05
      | -4.9749E-05
      | -1.7362E-06
      | 2.6691E-05
      | -4.4279E-05
      | -2.4363E-06
      | 3.9821E-05
      | -4.1687E-05
      | 5.3371E-07
      | 4.3082E-05
      | -4.2289E-05
      | -4.5361E-07
      | 4.1207E-05
      | -4.2616E-05
      | -4.5361E-07
      | 4.0204E-05
      | -4.2521E-05
      | -1.6159E-06
      | 3.9463E-05
      | ],[3,4,3])
      settings: InputPortMap=u0,u1,u2
  KdX4 : Lookup_n-D  NumberOfTableDimensions=3  BreakpointsForDimension1=[-10 0 10]  BreakpointsForDimension2=|  BreakpointsForDimension3=[-5.14444 -3.08666664 -1.54332]  Table=|  InternalRulePriority=Speed  RndMeth=Simplest
      BreakpointsForDimension2=|
      | [-36.4062987
      | -18.4062987
      | -15.4062987
      | -13.9062987]
      Table=|
      | reshape([-4.0969E-05
      | -4.5313E-07
      | 4.0019E-05
      | -4.1787E-05
      | -1.2714E-06
      | 3.9006E-05
      | -4.8908E-05
      | -1.2714E-06
      | 3.0663E-05
      | -4.2681E-05
      | -2.1920E-06
      | 3.7920E-05
      | -4.0777E-05
      | -3.6185E-07
      | 4.0047E-05
      | -4.1470E-05
      | -1.0577E-06
      | 3.9147E-05
      | -4.8908E-05
      | -1.4679E-06
      | 3.0663E-05
      | -4.2187E-05
      | -1.7779E-06
      | 3.8312E-05
      | -4.0496E-05
      | -2.8854E-07
      | 4.0049E-05
      | -4.1082E-05
      | -9.2714E-07
      | 3.9223E-05
      | -4.1472E-05
      | -9.2714E-07
      | 3.8784E-05
      | -4.1733E-05
      | -1.5768E-06
      | 3.8383E-05
      | ],[3,4,3])
      settings: InputPortMap=u0,u1,u2
  Mux : Mux
  Selector1 : Selector  InputPortWidth=5  IndexOptions=Index vector (dialog)  Indices=2  OutputSizes=1
  Selector2 : Selector  InputPortWidth=5  IndexOptions=Index vector (dialog)  Indices=3  OutputSizes=1
  Selector3 : Selector  InputPortWidth=5  IndexOptions=Index vector (dialog)  Indices=4  OutputSizes=1
  Selector4 : Selector  InputPortWidth=5  IndexOptions=Index vector (dialog)  Indices=1  OutputSizes=1
  Selector5 : Selector  InputPortWidth=5  IndexOptions=Index vector (dialog)  Indices=2  OutputSizes=1
  Selector6 : Selector  InputPortWidth=5  IndexOptions=Index vector (dialog)  Indices=3  OutputSizes=1
  Selector7 : Selector  InputPortWidth=5  IndexOptions=Index vector (dialog)  Indices=1  OutputSizes=1
  Selector8 : Selector  InputPortWidth=5  IndexOptions=Index vector (dialog)  Indices=4  OutputSizes=1
  KdXi : Outport
  wires:
  Selector5/1 -> KdX2/3
  Selector6/1 -> KdX3/3
  Selector8/1 -> KdX4/3
  Selector4/1 -> KdX1/3
  UeX/1 -> Selector4/1, Selector5/1, Selector8/1, Selector6/1
  Selector3/1 -> KdX4/1
  Selector2/1 -> KdX3/1
  Selector1/1 -> KdX2/1
  KdX4/1 -> Mux/4
  KdX3/1 -> Mux/3
  KdX2/1 -> Mux/2
  KdX1/1 -> Mux/1
  z/1 -> KdX1/2, KdX2/2, KdX3/2, KdX4/2
  Mux/1 -> KdXi/1
  Selector7/1 -> KdX1/1
  dX/1 -> Selector7/1, Selector2/1, Selector3/1, Selector1/1

== system ctrl_TT_ad_ctrl_cpp_ros_feedback/HDM/HDM B3/M/Mdxi ==
  dX : Inport
  z : Inport  Port=2
  Demux6 : Demux  Outputs=5
  Gain{,1..4} (5 alike) : Gain
  Mux : Mux  Inputs=5
  ZudX1 q+1 : Lookup_n-D  BreakpointsForDimension1=[-30 -20 -10 0 10 20 30]  BreakpointsForDimension2=[-35.0624 -15.3724 -13.8724]  BreakpointsForDimension3=[-5.14444 -3.08666664 -1.54332]  Table=|  InternalRulePriority=Speed  RndMeth=Simplest
      | reshape([0.000594819
      | 0.000394915
      | 0.000195011
      | -4.89222E-06
      | -0.000204796
      | -0.0004047
      | -0.000604603
      | 0.000596203
      | 0.000392018
      | 0.000187833
      | -1.6352E-05
      | -0.000220537
      | -0.000424722
      | -0.000628907
      | 0.000582351
      | 0.000381446
      | 0.000180542
      | -2.03625E-05
      | -0.000221267
      | -0.000422171
      | -0.000623076
      | ],[7,3])
      settings: InputPortMap=u0,u1
  ZudX1 q+2 : Lookup_n-D  BreakpointsForDimension1=[-30 -20 -10 0 10 20 30]  BreakpointsForDimension2=[-35.0624 -15.3724 -13.8724]  BreakpointsForDimension3=[-5.14444 -3.08666664 -1.54332]  Table=|  InternalRulePriority=Speed  RndMeth=Simplest
      | reshape([0.000583784
      | 0.000394316
      | 0.000204847
      | 1.53782E-05
      | -0.000174091
      | -0.000363559
      | -0.000553028
      | 0.00056228
      | 0.000374724
      | 0.000187169
      | -3.86644E-07
      | -0.000187942
      | -0.000375498
      | -0.000563053
      | 0.000546298
      | 0.000362052
      | 0.000177806
      | -6.43933E-06
      | -0.000190685
      | -0.000374931
      | -0.000559176],[7,3])
      settings: InputPortMap=u0,u1
  ZudX1 q+3 : Lookup_n-D  BreakpointsForDimension1=[-30 -20 -10 0 10 20 30]  BreakpointsForDimension2=[-35.0624 -15.3724 -13.8724]  BreakpointsForDimension3=[-5.14444 -3.08666664 -1.54332]  Table=|  InternalRulePriority=Speed  RndMeth=Simplest
      | reshape([-0.000586989
      | -0.000395541
      | -0.000204094
      | -1.26467E-05
      | 0.000178801
      | 0.000370248
      | 0.000561695
      | -0.000568868
      | -0.000379268
      | -0.000189669
      | -6.86388E-08
      | 0.000189531
      | 0.000379131
      | 0.000568731
      | -0.000565299
      | -0.000378949
      | -0.000192598
      | -6.24776E-06
      | 0.000180103
      | 0.000366453
      | 0.000552804],[7,3])
      settings: InputPortMap=u0,u1
  ZudX1 q+4 : Lookup_n-D  BreakpointsForDimension1=[-30 -20 -10 0 10 20 30]  BreakpointsForDimension2=[-35.0624 -15.3724 -13.8724]  BreakpointsForDimension3=[-5.14444 -3.08666664 -1.54332]  Table=|  InternalRulePriority=Speed  RndMeth=Simplest
      | reshape([-0.000638396
      | -0.000426715
      | -0.000215035
      | -3.35454E-06
      | 0.000208326
      | 0.000420006
      | 0.000631687
      | -0.000598951
      | -0.000393944
      | -0.000188937
      | 1.60698E-05
      | 0.000221077
      | 0.000426084
      | 0.000631091
      | -0.000622514
      | -0.000421726
      | -0.000220939
      | -2.01522E-05
      | 0.000180635
      | 0.000381422
      | 0.000582209],[7,3])
      settings: InputPortMap=u0,u1
  ZudX1 q+5 : Lookup_n-D  BreakpointsForDimension1=[-30 -20 -10 0 10 20 30]  BreakpointsForDimension2=[-35.0624 -15.3724 -13.8724]  BreakpointsForDimension3=[-35.0624 -15.3724 -13.8724]  Table=|  InternalRulePriority=Speed  RndMeth=Simplest
      | reshape([-0.000461714
      | -0.000296336
      | -0.000130959
      | 3.44194E-05
      | 0.000199797
      | 0.000365175
      | 0.000530553
      | -0.000503641
      | -0.000327652
      | -0.000151663
      | 2.43257E-05
      | 0.000200315
      | 0.000376303
      | 0.000552292
      | -0.000536558
      | -0.000356664
      | -0.00017677
      | 3.1235E-06
      | 0.000183017
      | 0.000362911
      | 0.000542805],[7,3])
      settings: InputPortMap=u0,u1
  MdX : Outport
  wires:
  Gain4/1 -> Mux/5
  Gain1/1 -> Mux/4
  Gain2/1 -> Mux/3
  Gain3/1 -> Mux/2
  Gain/1 -> Mux/1
  dX/1 -> Demux6/1
  Demux6/1 -> ZudX1 q+1/1
  Mux/1 -> MdX/1
  z/1 -> ZudX1 q+1/2, ZudX1 q+2/2, ZudX1 q+3/2, ZudX1 q+4/2, ZudX1 q+5/2
  ZudX1 q+5/1 -> Gain4/1
  ZudX1 q+1/1 -> Gain/1
  ZudX1 q+2/1 -> Gain3/1
  ZudX1 q+3/1 -> Gain2/1
  ZudX1 q+4/1 -> Gain1/1
  Demux6/2 -> ZudX1 q+2/1
  Demux6/3 -> ZudX1 q+3/1
  Demux6/4 -> ZudX1 q+4/1
  Demux6/5 -> ZudX1 q+5/1

== system ctrl_TT_ad_ctrl_cpp_ros_feedback/HDM/HDM B3/N/NdXi ==
  dX : Inport
  z : Inport  Port=2
  Mux : Mux
  NdX1 : Lookup_n-D  BreakpointsForDimension1=[-10 0 10]  BreakpointsForDimension2=|  BreakpointsForDimension3=[-5.14444 -3.08666664 -1.54332]  Table=|  InternalRulePriority=Speed  RndMeth=Simplest
      BreakpointsForDimension2=|
      | [-36.4062987
      | -18.4062987
      | -15.4062987
      | -13.9062987]
      Table=|
      | reshape([-8.13475E-05
      | -3.25752E-06
      | 6.9363E-05
      | -8.00129E-05
      | -1.7093E-06
      | 7.14001E-05
      | -6.46417E-05
      | -1.7093E-06
      | 8.57128E-05
      | -7.85432E-05
      | -1.19372E-08
      | 7.37459E-05],[3,4])
      settings: InputPortMap=u0,u1
  NdX2 : Lookup_n-D  BreakpointsForDimension1=[-10 0 10]  BreakpointsForDimension2=|  BreakpointsForDimension3=[-5.14444 -3.08666664 -1.54332]  Table=|  InternalRulePriority=Speed  RndMeth=Simplest
      BreakpointsForDimension2=|
      | [-36.4062987
      | -18.4062987
      | -15.4062987
      | -13.9062987]
      Table=|
      | reshape([6.2278E-05
      | -3.5277E-06
      | -7.1028E-05
      | 5.9473E-05
      | -6.2352E-06
      | -7.5067E-05
      | 3.9525E-05
      | -6.2352E-06
      | -9.4282E-05
      | 5.5892E-05
      | -1.0640E-05
      | -8.2654E-05],[3,4])
      settings: InputPortMap=u0,u1
  NdX3 : Lookup_n-D  BreakpointsForDimension1=[-10 0 10]  BreakpointsForDimension2=|  BreakpointsForDimension3=[-5.14444 -3.08666664 -1.54332]  Table=|  InternalRulePriority=Speed  RndMeth=Simplest
      BreakpointsForDimension2=|
      | [-36.4062987
      | -18.4062987
      | -15.4062987
      | -13.9062987]
      Table=|
      | reshape([8.96891E-05
      | 3.65995E-06
      | -8.07998E-05
      | 9.13096E-05
      | 6.34009E-06
      | -7.59117E-05
      | 0.000100356
      | 6.34009E-06
      | -4.56822E-05
      | 9.40576E-05
      | 1.06795E-05
      | -6.79415E-05],[3,4])
      settings: InputPortMap=u0,u1
  NdX4 : Lookup_n-D  BreakpointsForDimension1=[-10 0 10]  BreakpointsForDimension2=|  BreakpointsForDimension3=[-5.14444 -3.08666664 -1.54332]  Table=|  InternalRulePriority=Speed  RndMeth=Simplest
      BreakpointsForDimension2=|
      | [-36.4062987
      | -18.4062987
      | -15.4062987
      | -13.9062987]
      Table=|
      | reshape([-7.16232E-05
      | 3.25314E-06
      | 8.32589E-05
      | -7.3213E-05
      | 1.68586E-06
      | 8.13825E-05
      | -8.66615E-05
      | 1.68586E-06
      | 6.54218E-05
      | -7.48528E-05
      | -6.7812E-08
      | 7.92559E-05],[3,4])
      settings: InputPortMap=u0,u1
  Selector1 : Selector  InputPortWidth=5  IndexOptions=Index vector (dialog)  Indices=2  OutputSizes=1
  Selector2 : Selector  InputPortWidth=5  IndexOptions=Index vector (dialog)  Indices=3  OutputSizes=1
  Selector3 : Selector  InputPortWidth=5  IndexOptions=Index vector (dialog)  Indices=4  OutputSizes=1
  Selector7 : Selector  InputPortWidth=5  IndexOptions=Index vector (dialog)  Indices=1  OutputSizes=1
  NdXi : Outport
  wires:
  Selector3/1 -> NdX4/1
  Selector2/1 -> NdX3/1
  Selector1/1 -> NdX2/1
  NdX4/1 -> Mux/4
  NdX3/1 -> Mux/3
  NdX2/1 -> Mux/2
  NdX1/1 -> Mux/1
  z/1 -> NdX1/2, NdX2/2, NdX3/2, NdX4/2
  Mux/1 -> NdXi/1
  Selector7/1 -> NdX1/1
  dX/1 -> Selector7/1, Selector1/1, Selector2/1, Selector3/1
